simulink library "xpclib"  (Simulink 6.0)
settings: Solver=ode45  SolverMode=SingleTasking  StartTime=0.0  StopTime=10.0  RelTol=1e-3
values from neighbouring files (symbols this model uses):
  base = get_param( gcb, 'base' )    [maddiamondmm.m]    (also in maddiamondmm32frame.m; maddsmm16at.m; mdadsmm16at.m; mdiortddm64x0.m = hex2dec(addr(3:end)))
  block = find_system(bdroot,                          'FollowLinks', 'on',                          'LookUnderMasks', 'all',                          'MaskType', type )    [mdionipci6527.m]
  count = count + 1    (= 5)    [mdecodestate.m]
  port = get_param( gcb, 'port' )    [mdionipci6527.m]    (also in mdiortddm64x0.m = get_param(blocks{i}, 'port'))
undefined symbols (not defined in the file or in its folder): CIO, devid, DIO24, genixlib, get, handlers, irq, mbaseserialmask, mbwaudpmc, mdacbpcidas, mdiamondemeraldmask, mgenix, mmodemcontrol, mquamask, mrs232, msc150checks, mtargetboxleds, mtargetboxwatchdog, mxpccan, PCI, sizeof, vendid
libraries: xpclib x384, simulink x6
(part 1 of 7)
settings Model: RequirementInfo=9  CovMetricSettings=d  Creator=mvetsch  LastModifiedBy=gweast  ProdHWDeviceType=Specified  xpc_rtwmakecfg_data=_xpcaudpmc_
settings Model: ForwardingTableString=|
  | ||__slOldName__||xpclib/A//D/Advantech/PCL-1800 ||__slNewName__||xpcadvantechlib/A//D/PCL-1800 ||__slOldName__||xpclib/A//D/Advantech/PCL-711B||__slNewName__||xpcadvantechlib/A//D/PCL-711B||__slOldName__||xpclib/A//D/Advantech/PCL-812||__slNewName__||xpcadvantechlib/A//D/PCL-812||__slOldName__||xpclib/A//D/Advantech/PCL-812PG||__slNewName__||xpcadvantechlib/A//D/PCL-812PG||__slOldName__||xpclib/A//D/Advantech/PCL-818 ||__slNewName__||xpcadvantechlib/A//D/PCL-818 ||__slOldName__||xpclib/A//D/Advantech/PCL-818H ||__slNewName__||xpcadvantechlib/A//D/PCL-818H ||__slOldName__||xpclib/A//D/Advantech/PCL-818HD ||__slNewName__||xpcadvantechlib/A//D/PCL-818HD ||__slOldName__||xpclib/A//D/Advantech/PCL-818HG ||__slNewName__||xpcadvantechlib/A//D/PCL-818HG ||__slOldName__||xpclib/A//D/Advantech/PCL-818L ||__slNewName__||xpcadvantechlib/A//D/PCL-818L ||__slOldName__||xpclib/A//D/Analogic/AIM12 ||__slNewName__||xpcanalogiclib/A//D/AIM12 ||__slOldName__||xpclib/A//D/Analogic/AIM16 ||__slNewName__||xpcanalogiclib/A//D/AIM16 ||__slOldName__||xpclib/A//D/Burr-Brown/PCI-20019M ||__slNewName__||xpcobsoletelib/Burr-Brown/A//D/PCI-20019M ||__slOldName__||xpclib/A//D/Burr-Brown/PCI-20023M ||__slNewName__||xpcobsoletelib/Burr-Brown/A//D/PCI-20023M ||__slOldName__||xpclib/A//D/Burr-Brown/PCI-20098C ||__slNewName__||xpcobsoletelib/Burr-Brown/A//D/PCI-20098C ||__slOldName__||xpclib/A//D/Computer
  | Boards/CIO-DAS16 JR ||__slNewName__||xpcmeasurementcomputinglib/A//D/CIO-DAS16 JR ||__slOldName__||xpclib/A//D/Computer
  | Boards/CIO-DAS1601 12 ||__slNewName__||xpcmeasurementcomputinglib/A//D/CIO-DAS1601 12 ||__slOldName__||xpclib/A//D/Computer
  | Boards/CIO-DAS1602 12 ||__slNewName__||xpcmeasurementcomputinglib/A//D/CIO-DAS1602 12 ||__slOldName__||xpclib/A//D/Computer
  | Boards/CIO-DAS16 330 ||__slNewName__||xpcmeasurementcomputinglib/A//D/CIO-DAS16 330 ||__slOldName__||xpclib/A//D/Computer
  | Boards/CIO-DAS16JR EXP ||__slNewName__||xpcmeasurementcomputinglib/A//D/CIO-DAS16JR EXP ||__slOldName__||xpclib/A//D/Computer
  | Boards/CIO-DAS16JR 16 ||__slNewName__||xpcmeasurementcomputinglib/A//D/CIO-DAS16JR 16 ||__slOldName__||xpclib/A//D/Computer
  | Boards/CIO-DAS1602 16 ||__slNewName__||xpcmeasurementcomputinglib/A//D/CIO-DAS1602 16 ||__slOldName__||xpclib/A//D/Computer
  | Boards/PC104-DAS16JR 12 ||__slNewName__||xpcmeasurementcomputinglib/A//D/PC104-DAS16JR 12 ||__slOldName__||xpclib/A//D/Computer
  | Boards/PC104-DAS16JR 16 ||__slNewName__||xpcmeasurementcomputinglib/A//D/PC104-DAS16JR 16 ||__slOldName__||xpclib/A//D/Computer
  | Boards/PCI-DAS1200 JR ||__slNewName__||xpcmeasurementcomputinglib/A//D/PCI-DAS1200 JR ||__slOldName__||xpclib/A//D/Computer
  | Boards/PCI-DAS1200 ||__slNewName__||xpcmeasurementcomputinglib/A//D/PCI-DAS1200 ||__slOldName__||xpclib/A//D/Computer
  | Boards/PCI-DAS1602 12 ||__slNewName__||xpcmeasurementcomputinglib/A//D/PCI-DAS1602 12 ||__slOldName__||xpclib/A//D/Computer
  | Boards/PCI-DAS1602 16 ||__slNewName__||xpcmeasurementcomputinglib/A//D/PCI-DAS1602 16 ||__slOldName__||xpclib/A//D/Computer
  | Boards/PCIM-DAS1602 16 ||__slNewName__||xpcmeasurementcomputinglib/A//D/PCIM-DAS1602 16 ||__slOldName__||xpclib/A//D/Contec/AD12-16 ||__slNewName__||xpcconteclib/A//D/AD12-16 ||__slOldName__||xpclib/A//D/Contec/AD12-16E ||__slNewName__||xpcconteclib/A//D/AD12-16E ||__slOldName__||xpclib/A//D/Contec/AD12-16UE ||__slNewName__||xpcconteclib/A//D/AD12-16UE ||__slOldName__||xpclib/A//D/Contec/AD12-64 ||__slNewName__||xpcconteclib/A//D/AD12-64 ||__slOldName__||xpclib/A//D/Contec/AD16-16E ||__slNewName__||xpcconteclib/A//D/AD16-16E ||__slOldName__||xpclib/A//D/Data
  | Translation/DT2821 ||__slNewName__||xpcdatatranslationlib/A//D/DT2821 ||__slOldName__||xpclib/A//D/Data
  | Translation/DT2821-F-16SE ||__slNewName__||xpcdatatranslationlib/A//D/DT2821-F-16SE ||__slOldName__||xpclib/A//D/Data
  | Translation/DT2821-F-8DI ||__slNewName__||xpcdatatranslationlib/A//D/DT2821-F-8DI ||__slOldName__||xpclib/A//D/Data
  | Translation/DT2821-G-16SE ||__slNewName__||xpcdatatranslationlib/A//D/DT2821-G-16SE ||__slOldName__||xpclib/A//D/Data
  | Translation/DT2821-G-8DI ||__slNewName__||xpcdatatranslationlib/A//D/DT2821-G-8DI ||__slOldName__||xpclib/A//D/Data
  | Translation/DT2823 ||__slNewName__||xpcdatatranslationlib/A//D/DT2823 ||__slOldName__||xpclib/A//D/Data
  | Translation/DT2824-PGH ||__slNewName__||xpcdatatranslationlib/A//D/DT2824-PGH ||__slOldName__||xpclib/A//D/Data
  | Translation/DT2824-PGL ||__slNewName__||xpcdatatranslationlib/A//D/DT2824-PGL ||__slOldName__||xpclib/A//D/Data
  | Translation/DT2825 ||__slNewName__||xpcdatatranslationlib/A//D/DT2825 ||__slOldName__||xpclib/A//D/Data
  | Translation/DT2827 ||__slNewName__||xpcdatatranslationlib/A//D/DT2827 ||__slOldName__||xpclib/A//D/Data
  | Translation/DT2828 ||__slNewName__||xpcdatatranslationlib/A//D/DT2828 ||__slOldName__||xpclib/A//D/Diamond/MM ||__slNewName__||xpcdiamondlib/A//D/MM ||__slOldName__||xpclib/A//D/Diamond/MM-16-AT ||__slNewName__||xpcdiamondlib/A//D/MM-16-AT ||__slOldName__||xpclib/A//D/Diamond/MM-32 ||__slNewName__||xpcdiamondlib/A//D/MM-32 ||__slOldName__||xpclib/A//D/Diamond/Prometheus ||__slNewName__||xpcdiamondlib/A//D/Prometheus ||__slOldName__||xpclib/A//D/General
  | Standards/ADADIO ||__slNewName__||xpcgeneralstandardslib/A//D/ADADIO ||__slOldName__||xpclib/A//D/General
  | Standards/ADADIO 1||__slNewName__||xpcgeneralstandardslib/A//D/ADADIO 1||__slOldName__||xpclib/A//D/General
  | Standards/Create Enable Signal||__slNewName__||xpcgeneralstandardslib/A//D/Create Enable Signal||__slOldName__||xpclib/A//D/Gespac/GESADA-1 ||__slNewName__||xpcobsoletelib/Gespac/A//D/GESADA-1 ||__slOldName__||xpclib/A//D/Humusoft/AD 512 ||__slNewName__||xpchumusoftlib/A//D/AD 512 ||__slOldName__||xpclib/A//D/Keithley
  | Metrabyte/KPCI-1801HC ||__slNewName__||xpckeithleylib/A//D/KPCI-1801HC ||__slOldName__||xpclib/A//D/Keithley
  | Metrabyte/KPCI-1802HC ||__slNewName__||xpckeithleylib/A//D/KPCI-1802HC ||__slOldName__||xpclib/A//D/Keithley
  | Metrabyte/DAS-1800HR ||__slNewName__||xpckeithleylib/A//D/DAS-1800HR ||__slOldName__||xpclib/A//D/National
  | Instruments/PCI-6023E ||__slNewName__||xpcnilib/A//D/PCI-6023E ||__slOldName__||xpclib/A//D/National
  | Instruments/PCI-6024E ||__slNewName__||xpcnilib/A//D/PCI-6024E ||__slOldName__||xpclib/A//D/National
  | Instruments/PCI-6025E ||__slNewName__||xpcnilib/A//D/PCI-6025E ||__slOldName__||xpclib/A//D/National
  | Instruments/PCI-6031E ||__slNewName__||xpcnilib/A//D/PCI-6031E ||__slOldName__||xpclib/A//D/National
  | Instruments/PCI-6052E ||__slNewName__||xpcnilib/A//D/PCI-6052E ||__slOldName__||xpclib/A//D/National
  | Instruments/PCI-6071E ||__slNewName__||xpcnilib/A//D/PCI-6071E ||__slOldName__||xpclib/A//D/National
  | Instruments/PCI-MIO-16E-1 ||__slNewName__||xpcnilib/A//D/PCI-6070E ||__slOldName__||xpclib/A//D/National
  | Instruments/PCI-MIO-16E-4 ||__slNewName__||xpcnilib/A//D/PCI-6040E ||__slOldName__||xpclib/A//D/National
  | Instruments/PCI-MIO-16XE-10 ||__slNewName__||xpcnilib/A//D/PCI-6030E ||__slOldName__||xpclib/A//D/National
  | Instruments/PXI-6040E ||__slNewName__||xpcnilib/A//D/PXI-6040E ||__slOldName__||xpclib/A//D/National
  | Instruments/PXI-6070E ||__slNewName__||xpcnilib/A//D/PXI-6070E ||__slOldName__||xpclib/A//D/National
  | Instruments/PXI-6071E ||__slNewName__||xpcnilib/A//D/PXI-6071E ||__slOldName__||xpclib/A//D/Quanser/Q8 ||__slNewName__||xpcquanserlib/A//D/Q8 ||__slOldName__||xpclib/A//D/Real Time
  | Devices/DM6420 ||__slNewName__||xpcrealtimedeviceslib/A//D/DM6420 ||__slOldName__||xpclib/A//D/Real Time
  | Devices/DM6430 ||__slNewName__||xpcrealtimedeviceslib/A//D/DM6430 ||__slOldName__||xpclib/A//D/Real Time
  | Devices/DM7420 ||__slNewName__||xpcrealtimedeviceslib/A//D/DM7420 ||__slOldName__||xpclib/A//D/SBS
  | Technologies/IP-16ADC ||__slNewName__||xpcsbstechnologieslib/A//D/IP-16ADC ||__slOldName__||xpclib/A//D/SBS
  | Technologies/IP-HiADC ||__slNewName__||xpcsbstechnologieslib/A//D/IP-HiADC ||__slOldName__||xpclib/A//D/UEI/PD2-MF 12bit series ||__slNewName__||xpcueilib/A//D/PD2-MF 12bit series ||__slOldName__||xpclib/A//D/UEI/PD2-MF 14bit series ||__slNewName__||xpcueilib/A//D/PD2-MF 14bit series ||__slOldName__||xpclib/A//D/UEI/PD2-MF 16bit series ||__slNewName__||xpcueilib/A//D/PD2-MF 16bit series ||__slOldName__||xpclib/A//D/UEI/PD2-MFS 12bit series ||__slNewName__||xpcueilib/A//D/PD2-MFS 12bit series ||__slOldName__||xpclib/A//D/UEI/PD2-MFS 14bit series ||__slNewName__||xpcueilib/A//D/PD2-MFS 14bit series ||__slOldName__||xpclib/A//D/UEI/PD2-MFS 16bit series ||__slNewName__||xpcueilib/A//D/PD2-MFS 16bit series ||__slOldName__||xpclib/A//D/UEI/PDXI-MF 12bit series ||__slNewName__||xpcueilib/A//D/PDXI-MF 12bit series ||__slOldName__||xpclib/A//D/UEI/PDXI-MF 14bit series ||__slNewName__||xpcueilib/A//D/PDXI-MF 14bit series ||__slOldName__||xpclib/A//D/UEI/PDXI-MF 16bit series ||__slNewName__||xpcueilib/A//D/PDXI-MF 16bit series ||__slOldName__||xpclib/A//D/UEI/PDXI-MFS 12bit series ||__slNewName__||xpcueilib/A//D/PDXI-MFS 12bit series ||__slOldName__||xpclib/A//D/UEI/PDXI-MFS 14bit series ||__slNewName__||xpcueilib/A//D/PDXI-MFS 14bit series ||__slOldName__||xpclib/A//D/UEI/PDXI-MFS 16bit series ||__slNewName__||xpcueilib/A//D/PDXI-MFS 16bit series ||__slOldName__||xpclib/A//D/Versalogic/VSBC-6 ||__slNewName__||xpcversalogiclib/A//D/VSBC-6 ||__slOldName__||xpclib/A//D
  | Frame/Diamond/MM-32 Frame ||__slNewName__||xpcdiamondlib/A//D
  | Frame/MM-32 Frame ||__slOldName__||xpclib/A//D
  | Frame/UEI/PD2-MF Frame 12bit series ||__slNewName__||xpcueilib/A//D
  | Frame/PD2-MF Frame 12bit series ||__slOldName__||xpclib/A//D
  | Frame/UEI/PD2-MF Frame 14bit series ||__slNewName__||xpcueilib/A//D
  | Frame/PD2-MF Frame 14bit series ||__slOldName__||xpclib/A//D
  | Frame/UEI/PD2-MF Frame 16bit series ||__slNewName__||xpcueilib/A//D
  | Frame/PD2-MF Frame 16bit series ||__slOldName__||xpclib/A//D
  | Frame/UEI/PD2-MFS Frame 12bit series ||__slNewName__||xpcueilib/A//D
  | Frame/PD2-MFS Frame 12bit series ||__slOldName__||xpclib/A//D
  | Frame/UEI/PD2-MFS Frame 14bit series ||__slNewName__||xpcueilib/A//D
  | Frame/PD2-MFS Frame 14bit series ||__slOldName__||xpclib/A//D
  | Frame/UEI/PD2-MFS Frame 16bit series ||__slNewName__||xpcueilib/A//D
  | Frame/PD2-MFS Frame 16bit series ||__slOldName__||xpclib/A//D
  | Frame/UEI/PDXI-MF Frame 12bit series ||__slNewName__||xpcueilib/A//D
  | Frame/PDXI-MF Frame 12bit series ||__slOldName__||xpclib/A//D
  | Frame/UEI/PDXI-MF Frame 14bit series ||__slNewName__||xpcueilib/A//D
  | Frame/PDXI-MF Frame 14bit series ||__slOldName__||xpclib/A//D
  | Frame/UEI/PDXI-MF Frame 16bit series ||__slNewName__||xpcueilib/A//D
  | Frame/PDXI-MF Frame 16bit series ||__slOldName__||xpclib/A//D
  | Frame/UEI/PDXI-MFS Frame 12bit series ||__slNewName__||xpcueilib/A//D
  | Frame/PDXI-MFS Frame 12bit series ||__slOldName__||xpclib/A//D
  | Frame/UEI/PDXI-MFS Frame 14bit series ||__slNewName__||xpcueilib/A//D
  | Frame/PDXI-MFS Frame 14bit series ||__slOldName__||xpclib/A//D
  | Frame/UEI/PDXI-MFS Frame 16bit series ||__slNewName__||xpcueilib/A//D
  | Frame/PDXI-MFS Frame 16bit series ||__slOldName__||xpclib/D//A/Advantech/PCL-711B||__slNewName__||xpcadvantechlib/D//A/PCL-711B ||__slOldName__||xpclib/D//A/Advantech/PCL-812||__slNewName__||xpcadvantechlib/D//A/PCL-812 ||__slOldName__||xpclib/D//A/Advantech/PCL-812PG||__slNewName__||xpcadvantechlib/D//A/PCL-812PG ||__slOldName__||xpclib/D//A/Advantech/PCL-818 ||__slNewName__||xpcadvantechlib/D//A/PCL-818 ||__slOldName__||xpclib/D//A/Advantech/PCL-818L ||__slNewName__||xpcadvantechlib/D//A/PCL-818L ||__slOldName__||xpclib/D//A/Advantech/PCL-818HG ||__slNewName__||xpcadvantechlib/D//A/PCL-818HG ||__slOldName__||xpclib/D//A/Advantech/PCL-818H ||__slNewName__||xpcadvantechlib/D//A/PCL-818H ||__slOldName__||xpclib/D//A/Advantech/PCL-818HD ||__slNewName__||xpcadvantechlib/D//A/PCL-818HD ||__slOldName__||xpclib/D//A/Advantech/PCL-1800 ||__slNewName__||xpcadvantechlib/D//A/PCL-1800 ||__slOldName__||xpclib/D//A/Advantech/PCL-726 ||__slNewName__||xpcadvantechlib/D//A/PCL-726 ||__slOldName__||xpclib/D//A/Advantech/PCL-727 ||__slNewName__||xpcadvantechlib/D//A/PCL-727 ||__slOldName__||xpclib/D//A/Advantech/PCL-728 ||__slNewName__||xpcadvantechlib/D//A/PCL-728 ||__slOldName__||xpclib/D//A/Burr-Brown/PCI-20003M ||__slNewName__||xpcobsoletelib/Burr-Brown/D//A/PCI-20003M ||__slOldName__||xpclib/D//A/Computer
  | Boards/CIO-DAS1601 12 ||__slNewName__||xpcmeasurementcomputinglib/D//A/CIO-DAS1601 12 ||__slOldName__||xpclib/D//A/Computer
  | Boards/CIO-DAS1602 12 ||__slNewName__||xpcmeasurementcomputinglib/D//A/CIO-DAS1602 12 ||__slOldName__||xpclib/D//A/Computer
  | Boards/CIO-DAS1602 16 ||__slNewName__||xpcmeasurementcomputinglib/D//A/CIO-DAS1602 16 ||__slOldName__||xpclib/D//A/Computer
  | Boards/CIO-DDA06 ||__slNewName__||xpcmeasurementcomputinglib/D//A/CIO-DDA06 ||__slOldName__||xpclib/D//A/Computer
  | Boards/CIO-DAC08 ||__slNewName__||xpcmeasurementcomputinglib/D//A/CIO-DAC08 ||__slOldName__||xpclib/D//A/Computer
  | Boards/CIO-DAC16 ||__slNewName__||xpcmeasurementcomputinglib/D//A/CIO-DAC16 ||__slOldName__||xpclib/D//A/Computer
  | Boards/PC104-DAC06 ||__slNewName__||xpcmeasurementcomputinglib/D//A/PC104-DAC06 ||__slOldName__||xpclib/D//A/Computer
  | Boards/CIO-DDA06 16 ||__slNewName__||xpcmeasurementcomputinglib/D//A/CIO-DDA06 16 ||__slOldName__||xpclib/D//A/Computer
  | Boards/CIO-DAC08 16 ||__slNewName__||xpcmeasurementcomputinglib/D//A/CIO-DAC08 16 ||__slOldName__||xpclib/D//A/Computer
  | Boards/CIO-DAC16 16 ||__slNewName__||xpcmeasurementcomputinglib/D//A/CIO-DAC16 16 ||__slOldName__||xpclib/D//A/Computer
  | Boards/PCI-DAS1200 ||__slNewName__||xpcmeasurementcomputinglib/D//A/PCI-DAS1200 ||__slOldName__||xpclib/D//A/Computer
  | Boards/PCI-DAS1602 12 ||__slNewName__||xpcmeasurementcomputinglib/D//A/PCI-DAS1602 12 ||__slOldName__||xpclib/D//A/Computer
  | Boards/PCI-DAS1602 16 ||__slNewName__||xpcmeasurementcomputinglib/D//A/PCI-DAS1602 16 ||__slOldName__||xpclib/D//A/Computer
  | Boards/PCIM-DAS1602 16 ||__slNewName__||xpcmeasurementcomputinglib/D//A/PCIM-DAS1602 16 ||__slOldName__||xpclib/D//A/Computer
  | Boards/PCI-DDA02 12 ||__slNewName__||xpcmeasurementcomputinglib/D//A/PCI-DDA02 12 ||__slOldName__||xpclib/D//A/Computer
  | Boards/PCI-DDA04 12 ||__slNewName__||xpcmeasurementcomputinglib/D//A/PCI-DDA04 12 ||__slOldName__||xpclib/D//A/Computer
  | Boards/PCI-DDA08 12 ||__slNewName__||xpcmeasurementcomputinglib/D//A/PCI-DDA08 12 ||__slOldName__||xpclib/D//A/Computer
  | Boards/PCI-DDA02 16 ||__slNewName__||xpcmeasurementcomputinglib/D//A/PCI-DDA02 16 ||__slOldName__||xpclib/D//A/Computer
  | Boards/PCI-DDA04 16 ||__slNewName__||xpcmeasurementcomputinglib/D//A/PCI-DDA04 16 ||__slOldName__||xpclib/D//A/Computer
  | Boards/PCI-DDA08 16 ||__slNewName__||xpcmeasurementcomputinglib/D//A/PCI-DDA08 16 ||__slOldName__||xpclib/D//A/Computer
  | Boards/PCIM-DDA06 16 ||__slNewName__||xpcmeasurementcomputinglib/D//A/PCIM-DDA06 16 ||__slOldName__||xpclib/D//A/Contec/DA12-4 ||__slNewName__||xpcconteclib/D//A/DA12-4 ||__slOldName__||xpclib/D//A/Contec/DA12-16 ||__slNewName__||xpcconteclib/D//A/DA12-16 ||__slOldName__||xpclib/D//A/Contec/AD12-16E ||__slNewName__||xpcconteclib/D//A/AD12-16E ||__slOldName__||xpclib/D//A/Contec/AD12-16UE  ||__slNewName__||xpcconteclib/D//A/AD12-16UE ||__slOldName__||xpclib/D//A/Contec/AD16-16E  ||__slNewName__||xpcconteclib/D//A/AD16-16E ||__slOldName__||xpclib/D//A/Data
  | Translation/DT2821 ||__slNewName__||xpcdatatranslationlib/D//A/DT2821 ||__slOldName__||xpclib/D//A/Data
  | Translation/DT2821-F-16SE ||__slNewName__||xpcdatatranslationlib/D//A/DT2821-F-16SE ||__slOldName__||xpclib/D//A/Data
  | Translation/DT2821-F-8DI ||__slNewName__||xpcdatatranslationlib/D//A/DT2821-F-8DI ||__slOldName__||xpclib/D//A/Data
  | Translation/DT2821-G-16SE ||__slNewName__||xpcdatatranslationlib/D//A/DT2821-G-16SE ||__slOldName__||xpclib/D//A/Data
  | Translation/DT2821-G-8DI ||__slNewName__||xpcdatatranslationlib/D//A/DT2821-G-8DI ||__slOldName__||xpclib/D//A/Data
  | Translation/DT2823 ||__slNewName__||xpcdatatranslationlib/D//A/DT2823 ||__slOldName__||xpclib/D//A/Data
  | Translation/DT2825 ||__slNewName__||xpcdatatranslationlib/D//A/DT2825 ||__slOldName__||xpclib/D//A/Data
  | Translation/DT2827 ||__slNewName__||xpcdatatranslationlib/D//A/DT2827 ||__slOldName__||xpclib/D//A/Data
  | Translation/DT2828 ||__slNewName__||xpcdatatranslationlib/D//A/DT2828 ||__slOldName__||xpclib/D//A/Diamond/Ruby-MM ||__slNewName__||xpcdiamondlib/D//A/Ruby-MM ||__slOldName__||xpclib/D//A/Diamond/Ruby-MM-416 ||__slNewName__||xpcdiamondlib/D//A/Ruby-MM-416 ||__slOldName__||xpclib/D//A/Diamond/Ruby-MM-1612 ||__slNewName__||xpcdiamondlib/D//A/Ruby-MM-1612 ||__slOldName__||xpclib/D//A/Diamond/MM ||__slNewName__||xpcdiamondlib/D//A/MM ||__slOldName__||xpclib/D//A/Diamond/MM-32 ||__slNewName__||xpcdiamondlib/D//A/MM-32 ||__slOldName__||xpclib/D//A/Diamond/Prometheus ||__slNewName__||xpcdiamondlib/D//A/Prometheus ||__slOldName__||xpclib/D//A/Diamond/MM-16-AT ||__slNewName__||xpcdiamondlib/D//A/MM-16-AT ||__slOldName__||xpclib/D//A/General
  | Standards/ADADIO ||__slNewName__||xpcgeneralstandardslib/D//A/ADADIO ||__slOldName__||xpclib/D//A/General
  | Standards/Create Enable Signal||__slNewName__||xpcgeneralstandardslib/D//A/Create Enable Signal||__slOldName__||xpclib/D//A/General
  | Standards/ADADIO 1||__slNewName__||xpcgeneralstandardslib/D//A/ADADIO 1||__slOldName__||xpclib/D//A/General
  | Standards/PMC-16AO-12 ||__slNewName__||xpcgeneralstandardslib/D//A/PMC-16AO-12 ||__slOldName__||xpclib/D//A/Gespac/GESADA-1 ||__slNewName__||xpcobsoletelib/Gespac/D//A/GESADA-1 ||__slOldName__||xpclib/D//A/Humusoft/AD 512 ||__slNewName__||xpchumusoftlib/D//A/AD 512 ||__slOldName__||xpclib/D//A/Keithley
  | Metrabyte/KPCI-1801HC ||__slNewName__||xpckeithleylib/D//A/KPCI-1801HC ||__slOldName__||xpclib/D//A/Keithley
  | Metrabyte/KPCI-1802HC ||__slNewName__||xpckeithleylib/D//A/KPCI-1802HC ||__slOldName__||xpclib/D//A/National
  | Instruments/AT-AO-6 ||__slNewName__||xpcnilib/D//A/AT-AO-6 ||__slOldName__||xpclib/D//A/National
  | Instruments/AT-AO-10 ||__slNewName__||xpcnilib/D//A/AT-AO-10 ||__slOldName__||xpclib/D//A/National
  | Instruments/PCI-6703 ||__slNewName__||xpcnilib/D//A/PCI-6703 ||__slOldName__||xpclib/D//A/National
  | Instruments/PXI-6071E ||__slNewName__||xpcnilib/D//A/PXI-6071E ||__slOldName__||xpclib/D//A/National
  | Instruments/PCI-6024E ||__slNewName__||xpcnilib/D//A/PCI-6024E ||__slOldName__||xpclib/D//A/National
  | Instruments/PCI-6025E ||__slNewName__||xpcnilib/D//A/PCI-6025E ||__slOldName__||xpclib/D//A/National
  | Instruments/PCI-6704 ||__slNewName__||xpcnilib/D//A/PCI-6704 ||__slOldName__||xpclib/D//A/National
  | Instruments/PXI-6704 ||__slNewName__||xpcnilib/D//A/PXI-6704 ||__slOldName__||xpclib/D//A/National
  | Instruments/PCI-MIO-16E-1 ||__slNewName__||xpcnilib/D//A/PCI-6070E ||__slOldName__||xpclib/D//A/National
  | Instruments/PCI-MIO-16E-4 ||__slNewName__||xpcnilib/D//A/PCI-6040E ||__slOldName__||xpclib/D//A/National
  | Instruments/PXI-6070E ||__slNewName__||xpcnilib/D//A/PXI-6070E ||__slOldName__||xpclib/D//A/National
  | Instruments/PXI-6040E ||__slNewName__||xpcnilib/D//A/PXI-6040E ||__slOldName__||xpclib/D//A/National
  | Instruments/PCI-6071E ||__slNewName__||xpcnilib/D//A/PCI-6071E ||__slOldName__||xpclib/D//A/National
  | Instruments/PCI-6052E ||__slNewName__||xpcnilib/D//A/PCI-6052E ||__slOldName__||xpclib/D//A/National
  | Instruments/PCI-MIO-16XE-10 ||__slNewName__||xpcnilib/D//A/PCI-6030E ||__slOldName__||xpclib/D//A/National
  | Instruments/PCI-6031E ||__slNewName__||xpcnilib/D//A/PCI-6031E ||__slOldName__||xpclib/D//A/National
  | Instruments/PCI-6713 ||__slNewName__||xpcnilib/D//A/PCI-6713 ||__slOldName__||xpclib/D//A/National
  | Instruments/PXI-6713 ||__slNewName__||xpcnilib/D//A/PXI-6713 ||__slOldName__||xpclib/D//A/National
  | Instruments/PCI-6713 1||__slNewName__||xpcnilib/D//A/PCI-6713 1 ||__slOldName__||xpclib/D//A/Real Time
  | Devices/DM6420 ||__slNewName__||xpcrealtimedeviceslib/D//A/DM6420 ||__slOldName__||xpclib/D//A/Real Time
  | Devices/DM6430 ||__slNewName__||xpcrealtimedeviceslib/D//A/DM6430 ||__slOldName__||xpclib/D//A/Real Time
  | Devices/DM6604 ||__slNewName__||xpcrealtimedeviceslib/D//A/DM6604 ||__slOldName__||xpclib/D//A/SBS
  | Technologies/IP-DAC ||__slNewName__||xpcsbstechnologieslib/D//A/IP-DAC ||__slOldName__||xpclib/D//A/SBS
  | Technologies/IP-16DAC ||__slNewName__||xpcsbstechnologieslib/D//A/IP-16DAC ||__slOldName__||xpclib/D//A/UEI/PD2-MF 12bit series ||__slNewName__||xpcueilib/D//A/PD2-MF 12bit series||__slOldName__||xpclib/D//A/UEI/PD2-MFS 12bit series ||__slNewName__||xpcueilib/D//A/PD2-MFS 12bit series||__slOldName__||xpclib/D//A/UEI/PDXI-MF 12bit series ||__slNewName__||xpcueilib/D//A/PDXI-MF 12bit series||__slOldName__||xpclib/D//A/UEI/PDXI-MFS 12bit series ||__slNewName__||xpcueilib/D//A/PDXI-MFS 12bit series||__slOldName__||xpclib/D//A/UEI/PD2-MF 14bit series ||__slNewName__||xpcueilib/D//A/PD2-MF 14bit series||__slOldName__||xpclib/D//A/UEI/PD2-MFS 14bit series ||__slNewName__||xpcueilib/D//A/PD2-MFS 14bit series||__slOldName__||xpclib/D//A/UEI/PDXI-MF 14bit series ||__slNewName__||xpcueilib/D//A/PDXI-MF 14bit series||__slOldName__||xpclib/D//A/UEI/PDXI-MFS 14bit series ||__slNewName__||xpcueilib/D//A/PDXI-MFS 14bit series||__slOldName__||xpclib/D//A/UEI/PD2-MF 16bit series ||__slNewName__||xpcueilib/D//A/PD2-MF 16bit series||__slOldName__||xpclib/D//A/UEI/PD2-MFS 16bit series ||__slNewName__||xpcueilib/D//A/PD2-MFS 16bit series||__slOldName__||xpclib/D//A/UEI/PDXI-MF 16bit series ||__slNewName__||xpcueilib/D//A/PDXI-MF 16bit series||__slOldName__||xpclib/D//A/UEI/PDXI-MFS 16bit series ||__slNewName__||xpcueilib/D//A/PDXI-MFS 16bit series||__slOldName__||xpclib/D//A/UEI/PD2-AO series ||__slNewName__||xpcueilib/D//A/PD2-AO series||__slOldName__||xpclib/D//A/UEI/PDXI-AO series ||__slNewName__||xpcueilib/D//A/PDXI-AO series||__slOldName__||xpclib/Digital
  | Input/Advantech/PCL-711B||__slNewName__||xpcadvantechlib/Digital
  | Input/PCL-711B ||__slOldName__||xpclib/Digital
  | Input/Advantech/PCL-812||__slNewName__||xpcadvantechlib/Digital
  | Input/PCL-812 ||__slOldName__||xpclib/Digital
  | Input/Advantech/PCL-812PG||__slNewName__||xpcadvantechlib/Digital
  | Input/PCL-812PG ||__slOldName__||xpclib/Digital
  | Input/Advantech/PCL-818 ||__slNewName__||xpcadvantechlib/Digital
  | Input/PCL-818 ||__slOldName__||xpclib/Digital
  | Input/Advantech/PCL-818L ||__slNewName__||xpcadvantechlib/Digital
  | Input/PCL-818L ||__slOldName__||xpclib/Digital
  | Input/Advantech/PCL-818HG ||__slNewName__||xpcadvantechlib/Digital
  | Input/PCL-818HG ||__slOldName__||xpclib/Digital
  | Input/Advantech/PCL-818H ||__slNewName__||xpcadvantechlib/Digital
  | Input/PCL-818H ||__slOldName__||xpclib/Digital
  | Input/Advantech/PCL-818HD ||__slNewName__||xpcadvantechlib/Digital
  | Input/PCL-818HD ||__slOldName__||xpclib/Digital
  | Input/Advantech/PCL-1800 ||__slNewName__||xpcadvantechlib/Digital
  | Input/PCL-1800 ||__slOldName__||xpclib/Digital
  | Input/Advantech/PCL-726 ||__slNewName__||xpcadvantechlib/Digital
  | Input/PCL-726 ||__slOldName__||xpclib/Digital
  | Input/Advantech/PCL-727 ||__slNewName__||xpcadvantechlib/Digital
  | Input/PCL-727 ||__slOldName__||xpclib/Digital
  | Input/Analogic/AIM12 ||__slNewName__||xpcanalogiclib/Digital
  | Input/AIM12 ||__slOldName__||xpclib/Digital
  | Input/Analogic/AIM16 ||__slNewName__||xpcanalogiclib/Digital
  | Input/AIM16 ||__slOldName__||xpclib/Digital
  | Input/Burr-Brown/PCI-20041C ||__slNewName__||xpcobsoletelib/Burr-Brown/Digital
  | Input/PCI-20041C ||__slOldName__||xpclib/Digital
  | Input/Burr-Brown/PCI-20098C ||__slNewName__||xpcobsoletelib/Burr-Brown/Digital
  | Input/PCI-20098C ||__slOldName__||xpclib/Digital
  | Input/BVM/PMCDIO64 ||__slNewName__||xpcobsoletelib/BVM/Digital
  | Input/PMCDIO64 ||__slOldName__||xpclib/Digital
  | Input/Computer
  | Boards/CIO-DDA06 ||__slNewName__||xpcmeasurementcomputinglib/Digital
  | Input/CIO-DDA06 ||__slOldName__||xpclib/Digital
  | Input/Computer
  | Boards/CIO-DDA06//16 ||__slNewName__||xpcmeasurementcomputinglib/Digital
  | Input/CIO-DDA06//16 ||__slOldName__||xpclib/Digital
  | Input/Computer
  | Boards/CIO-DAS1601 12 ||__slNewName__||xpcmeasurementcomputinglib/Digital
  | Input/CIO-DAS1601 12 ||__slOldName__||xpclib/Digital
  | Input/Computer
  | Boards/CIO-DAS1602 12 ||__slNewName__||xpcmeasurementcomputinglib/Digital
  | Input/CIO-DAS1602 12 ||__slOldName__||xpclib/Digital
  | Input/Computer
  | Boards/CIO-DAS1602 16 ||__slNewName__||xpcmeasurementcomputinglib/Digital
  | Input/CIO-DAS1602 16 ||__slOldName__||xpclib/Digital
  | Input/Computer
  | Boards/CIO-DIO24 ||__slNewName__||xpcmeasurementcomputinglib/Digital
  | Input/CIO-DIO24 ||__slOldName__||xpclib/Digital
  | Input/Computer
  | Boards/CIO-DIO48 ||__slNewName__||xpcmeasurementcomputinglib/Digital
  | Input/CIO-DIO48 ||__slOldName__||xpclib/Digital
  | Input/Computer
  | Boards/CIO-DIO96 ||__slNewName__||xpcmeasurementcomputinglib/Digital
  | Input/CIO-DIO96 ||__slOldName__||xpclib/Digital
  | Input/Computer
  | Boards/CIO-DIO192 ||__slNewName__||xpcmeasurementcomputinglib/Digital
  | Input/CIO-DIO192 ||__slOldName__||xpclib/Digital
  | Input/Computer
  | Boards/CIO-DIO24H ||__slNewName__||xpcmeasurementcomputinglib/Digital
  | Input/CIO-DIO24H ||__slOldName__||xpclib/Digital
  | Input/Computer
  | Boards/CIO-DIO48H ||__slNewName__||xpcmeasurementcomputinglib/Digital
  | Input/CIO-DIO48H ||__slOldName__||xpclib/Digital
  | Input/Computer
  | Boards/CIO-PDISO16 ||__slNewName__||xpcmeasurementcomputinglib/Digital
  | Input/CIO-PDISO16 ||__slOldName__||xpclib/Digital
  | Input/Computer
  | Boards/PC104-DAS16JR 12 ||__slNewName__||xpcmeasurementcomputinglib/Digital
  | Input/PC104-DAS16JR 12 ||__slOldName__||xpclib/Digital
  | Input/Computer
  | Boards/PC104-DAS16JR 16 ||__slNewName__||xpcmeasurementcomputinglib/Digital
  | Input/PC104-DAS16JR 16 ||__slOldName__||xpclib/Digital
  | Input/Computer
  | Boards/PC104-DIO48 ||__slNewName__||xpcmeasurementcomputinglib/Digital
  | Input/PC104-DIO48 ||__slOldName__||xpclib/Digital
  | Input/Computer
  | Boards/PCI-DAS1200 ||__slNewName__||xpcmeasurementcomputinglib/Digital
  | Input/PCI-DAS1200 ||__slOldName__||xpclib/Digital
  | Input/Computer
  | Boards/PCI-DAS1200 JR ||__slNewName__||xpcmeasurementcomputinglib/Digital
  | Input/PCI-DAS1200 JR ||__slOldName__||xpclib/Digital
  | Input/Computer
  | Boards/PCI-DAS1602 12 ||__slNewName__||xpcmeasurementcomputinglib/Digital
  | Input/PCI-DAS1602 12 ||__slOldName__||xpclib/Digital
  | Input/Computer
  | Boards/PCI-DAS1602 16 ||__slNewName__||xpcmeasurementcomputinglib/Digital
  | Input/PCI-DAS1602 16 ||__slOldName__||xpclib/Digital
  | Input/Computer
  | Boards/PCIM-DAS1602 16 ||__slNewName__||xpcmeasurementcomputinglib/Digital
  | Input/PCIM-DAS1602 16 ||__slOldName__||xpclib/Digital
  | Input/Computer
  | Boards/PCI-DIO24 ||__slNewName__||xpcmeasurementcomputinglib/Digital
  | Input/PCI-DIO24 ||__slOldName__||xpclib/Digital
  | Input/Computer
  | Boards/PCI-DIO24H ||__slNewName__||xpcmeasurementcomputinglib/Digital
  | Input/PCI-DIO24H ||__slOldName__||xpclib/Digital
  | Input/Computer
  | Boards/PCI-DIO48H ||__slNewName__||xpcmeasurementcomputinglib/Digital
  | Input/PCI-DIO48H ||__slOldName__||xpclib/Digital
  | Input/Computer
  | Boards/PCI-DIO96 ||__slNewName__||xpcmeasurementcomputinglib/Digital
  | Input/PCI-DIO96 ||__slOldName__||xpclib/Digital
  | Input/Computer
  | Boards/PCI-DIO96H ||__slNewName__||xpcmeasurementcomputinglib/Digital
  | Input/PCI-DIO96H ||__slOldName__||xpclib/Digital
  | Input/Computer
  | Boards/PCI-DDA02 12 ||__slNewName__||xpcmeasurementcomputinglib/Digital
  | Input/PCI-DDA02 12 ||__slOldName__||xpclib/Digital
  | Input/Computer
  | Boards/PCI-DDA04 12 ||__slNewName__||xpcmeasurementcomputinglib/Digital
  | Input/PCI-DDA04 12 ||__slOldName__||xpclib/Digital
  | Input/Computer
  | Boards/PCI-DDA08 12 ||__slNewName__||xpcmeasurementcomputinglib/Digital
  | Input/PCI-DDA08 12 ||__slOldName__||xpclib/Digital
  | Input/Computer
  | Boards/PCI-PDISO8 ||__slNewName__||xpcmeasurementcomputinglib/Digital
  | Input/PCI-PDISO8 ||__slOldName__||xpclib/Digital
  | Input/Computer
  | Boards/PCI-PDISO16 ||__slNewName__||xpcmeasurementcomputinglib/Digital
  | Input/PCI-PDISO16 ||__slOldName__||xpclib/Digital
  | Input/Computer
  | Boards/PCI-DDA02 16 ||__slNewName__||xpcmeasurementcomputinglib/Digital
  | Input/PCI-DDA02 16 ||__slOldName__||xpclib/Digital
  | Input/Computer
  | Boards/PCI-DDA04 16 ||__slNewName__||xpcmeasurementcomputinglib/Digital
  | Input/PCI-DDA04 16 ||__slOldName__||xpclib/Digital
  | Input/Computer
  | Boards/PCI-DDA08 16 ||__slNewName__||xpcmeasurementcomputinglib/Digital
  | Input/PCI-DDA08 16 ||__slOldName__||xpclib/Digital
  | Input/Computer
  | Boards/PCIM-DDA06 16 ||__slNewName__||xpcmeasurementcomputinglib/Digital
  | Input/PCIM-DDA06 16 ||__slOldName__||xpclib/Digital
  | Input/Computer
  | Boards/PCI-DUAL-AC5 ||__slNewName__||xpcmeasurementcomputinglib/Digital
  | Input/PCI-DUAL-AC5 ||__slOldName__||xpclib/Digital
  | Input/Contec/PIO-3232T ||__slNewName__||xpcconteclib/Digital
  | Input/PIO-3232T ||__slOldName__||xpclib/Digital
  | Input/Contec/AD12-16  ||__slNewName__||xpcconteclib/Digital
  | Input/AD12-16 ||__slOldName__||xpclib/Digital
  | Input/Contec/AD12-64 ||__slNewName__||xpcconteclib/Digital
  | Input/AD12-64 ||__slOldName__||xpclib/Digital
  | Input/Data
  | Translation/DT2821 ||__slNewName__||xpcdatatranslationlib/Digital
  | Input/DT2821 ||__slOldName__||xpclib/Digital
  | Input/Data
  | Translation/DT2821-F-16SE ||__slNewName__||xpcdatatranslationlib/Digital
  | Input/DT2821-F-16SE ||__slOldName__||xpclib/Digital
  | Input/Data
  | Translation/DT2821-F-8DI ||__slNewName__||xpcdatatranslationlib/Digital
  | Input/DT2821-F-8DI ||__slOldName__||xpclib/Digital
  | Input/Data
  | Translation/DT2821-G-16SE ||__slNewName__||xpcdatatranslationlib/Digital
  | Input/DT2821-G-16SE ||__slOldName__||xpclib/Digital
  | Input/Data
  | Translation/DT2821-G-8DI ||__slNewName__||xpcdatatranslationlib/Digital
  | Input/DT2821-G-8DI ||__slOldName__||xpclib/Digital
  | Input/Data
  | Translation/DT2823 ||__slNewName__||xpcdatatranslationlib/Digital
  | Input/DT2823 ||__slOldName__||xpclib/Digital
  | Input/Data
  | Translation/DT2824-PGH ||__slNewName__||xpcdatatranslationlib/Digital
  | Input/DT2824-PGH ||__slOldName__||xpclib/Digital
  | Input/Data
  | Translation/DT2824-PGL ||__slNewName__||xpcdatatranslationlib/Digital
  | Input/DT2824-PGL ||__slOldName__||xpclib/Digital
  | Input/Data
  | Translation/DT2825 ||__slNewName__||xpcdatatranslationlib/Digital
  | Input/DT2825 ||__slOldName__||xpclib/Digital
  | Input/Data
  | Translation/DT2827 ||__slNewName__||xpcdatatranslationlib/Digital
  | Input/DT2827 ||__slOldName__||xpclib/Digital
  | Input/Data
  | Translation/DT2828 ||__slNewName__||xpcdatatranslationlib/Digital
  | Input/DT2828 ||__slOldName__||xpclib/Digital
  | Input/Diamond/Ruby-MM ||__slNewName__||xpcdiamondlib/Digital
  | Input/Ruby-MM ||__slOldName__||xpclib/Digital
  | Input/Diamond/Ruby-MM-416 ||__slNewName__||xpcdiamondlib/Digital
  | Input/Ruby-MM-416 ||__slOldName__||xpclib/Digital
  | Input/Diamond/Ruby-MM-1612 ||__slNewName__||xpcdiamondlib/Digital
  | Input/Ruby-MM-1612 ||__slOldName__||xpclib/Digital
  | Input/Diamond/QUARTZ-MM-5 ||__slNewName__||xpcdiamondlib/Digital
  | Input/QUARTZ-MM-5 ||__slOldName__||xpclib/Digital
  | Input/Diamond/QUARTZ-MM-10 ||__slNewName__||xpcdiamondlib/Digital
  | Input/QUARTZ-MM-10 ||__slOldName__||xpclib/Digital
  | Input/Diamond/Prometheus ||__slNewName__||xpcdiamondlib/Digital
  | Input/Prometheus||__slOldName__||xpclib/Digital
  | Input/Diamond/MM ||__slNewName__||xpcdiamondlib/Digital
  | Input/MM ||__slOldName__||xpclib/Digital
  | Input/Diamond/MM-32 ||__slNewName__||xpcdiamondlib/Digital
  | Input/MM-32 ||__slOldName__||xpclib/Digital
  | Input/Diamond/MM-16-AT ||__slNewName__||xpcdiamondlib/Digital
  | Input/MM-16-AT ||__slOldName__||xpclib/Digital
  | Input/Diamond/Onyx-MM ||__slNewName__||xpcdiamondlib/Digital
  | Input/Onyx-MM ||__slOldName__||xpclib/Digital
  | Input/Diamond/Onyx-MM-DIO ||__slNewName__||xpcdiamondlib/Digital
  | Input/Onyx-MM-DIO ||__slOldName__||xpclib/Digital
  | Input/Diamond/Garnet-MM ||__slNewName__||xpcdiamondlib/Digital
  | Input/Garnet-MM ||__slOldName__||xpclib/Digital
  | Input/General
  | Standards/ADADIO ||__slNewName__||xpcgeneralstandardslib/Digital
  | Input/ADADIO ||__slOldName__||xpclib/Digital
  | Input/Gespac/GESPIA-2A ||__slNewName__||xpcobsoletelib/Gespac/Digital
  | Input/GESPIA-2A ||__slOldName__||xpclib/Digital
  | Input/Humusoft/AD 512 ||__slNewName__||xpchumusoftlib/Digital
  | Input/AD 512 ||__slOldName__||xpclib/Digital
  | Input/Keithley
  | Metrabyte/KPCI-1801HC ||__slNewName__||xpckeithleylib/Digital
  | Input/KPCI-1801HC ||__slOldName__||xpclib/Digital
  | Input/Keithley
  | Metrabyte/KPCI-1802HC ||__slNewName__||xpckeithleylib/Digital
  | Input/KPCI-1802HC ||__slOldName__||xpclib/Digital
  | Input/Keithley
  | Metrabyte/DAS-1800HR ||__slNewName__||xpckeithleylib/Digital
  | Input/DAS-1800HR ||__slOldName__||xpclib/Digital
  | Input/National
  | Instruments/PC-DIO-24 ||__slNewName__||xpcnilib/Digital
  | Input/PC-DIO-24 ||__slOldName__||xpclib/Digital
  | Input/National
  | Instruments/PC-TIO-10 ||__slNewName__||xpcnilib/Digital
  | Input/PC-TIO-10 ||__slOldName__||xpclib/Digital
  | Input/National
  | Instruments/PCI-6503 ||__slNewName__||xpcnilib/Digital
  | Input/PCI-6503 ||__slOldName__||xpclib/Digital
  | Input/National
  | Instruments/PCI-DIO-96 ||__slNewName__||xpcnilib/Digital
  | Input/PCI-DIO-96 ||__slOldName__||xpclib/Digital
  | Input/National
  | Instruments/PCI-6023E ||__slNewName__||xpcnilib/Digital
  | Input/PCI-6023E ||__slOldName__||xpclib/Digital
  | Input/National
  | Instruments/PCI-6024E ||__slNewName__||xpcnilib/Digital
  | Input/PCI-6024E ||__slOldName__||xpclib/Digital
  | Input/National
  | Instruments/PCI-6025E ||__slNewName__||xpcnilib/Digital
  | Input/PCI-6025E ||__slOldName__||xpclib/Digital
  | Input/National
  | Instruments/PCI-6025E 8255 ||__slNewName__||xpcnilib/Digital
  | Input/PCI-6025E 8255 ||__slOldName__||xpclib/Digital
  | Input/National
  | Instruments/PCI-MIO-16E-1 ||__slNewName__||xpcnilib/Digital
  | Input/PCI-6070E ||__slOldName__||xpclib/Digital
  | Input/National
  | Instruments/PCI-MIO-16E-4 ||__slNewName__||xpcnilib/Digital
  | Input/PCI-6040E ||__slOldName__||xpclib/Digital
  | Input/National
  | Instruments/PCI-6071E ||__slNewName__||xpcnilib/Digital
  | Input/PCI-6071E ||__slOldName__||xpclib/Digital
  | Input/National
  | Instruments/PCI-6527 ||__slNewName__||xpcnilib/Digital
  | Input/PCI-6527 ||__slOldName__||xpclib/Digital
  | Input/National
  | Instruments/PCI-6052E ||__slNewName__||xpcnilib/Digital
  | Input/PCI-6052E ||__slOldName__||xpclib/Digital
  | Input/National
  | Instruments/PCI-MIO-16XE-10 ||__slNewName__||xpcnilib/Digital
  | Input/PCI-6030E ||__slOldName__||xpclib/Digital
  | Input/National
  | Instruments/PCI-6031E ||__slNewName__||xpcnilib/Digital
  | Input/PCI-6031E ||__slOldName__||xpclib/Digital
  | Input/National
  | Instruments/PXI-6527 ||__slNewName__||xpcnilib/Digital
  | Input/PXI-6527 ||__slOldName__||xpclib/Digital
  | Input/National
  | Instruments/PXI-6070E ||__slNewName__||xpcnilib/Digital
  | Input/PXI-6070E ||__slOldName__||xpclib/Digital
  | Input/National
  | Instruments/PXI-6040E ||__slNewName__||xpcnilib/Digital
  | Input/PXI-6040E ||__slOldName__||xpclib/Digital
  | Input/National
  | Instruments/PXI-6508 ||__slNewName__||xpcnilib/Digital
  | Input/PXI-6508 ||__slOldName__||xpclib/Digital
  | Input/National
  | Instruments/PXI-6071E ||__slNewName__||xpcnilib/Digital
  | Input/PXI-6071E ||__slOldName__||xpclib/Digital
  | Input/National
  | Instruments/PCI-6713 ||__slNewName__||xpcnilib/Digital
  | Input/PCI-6713 ||__slOldName__||xpclib/Digital
  | Input/National
  | Instruments/PXI-6713 ||__slNewName__||xpcnilib/Digital
  | Input/PXI-6713 ||__slOldName__||xpclib/Digital
  | Input/National
  | Instruments/PCI-6711 ||__slNewName__||xpcnilib/Digital
  | Input/PCI-6711 ||__slOldName__||xpclib/Digital
  | Input/Real Time
  | Devices/DM6420 ||__slNewName__||xpcrealtimedeviceslib/Digital
  | Input/DM6420 ||__slOldName__||xpclib/Digital
  | Input/Real Time
  | Devices/DM6430 ||__slNewName__||xpcrealtimedeviceslib/Digital
  | Input/DM6430 ||__slOldName__||xpclib/Digital
  | Input/Real Time
  | Devices/DM7420 ||__slNewName__||xpcrealtimedeviceslib/Digital
  | Input/DM7420 ||__slOldName__||xpclib/Digital
  | Input/Real Time
  | Devices/DM6604 ||__slNewName__||xpcrealtimedeviceslib/Digital
  | Input/DM6604 ||__slOldName__||xpclib/Digital
  | Input/Real Time
  | Devices/DM6804 ||__slNewName__||xpcrealtimedeviceslib/Digital
  | Input/DM6804 ||__slOldName__||xpclib/Digital
  | Input/Real Time
  | Devices/DM6814 ||__slNewName__||xpcrealtimedeviceslib/Digital
  | Input/DM6814 ||__slOldName__||xpclib/Digital
  | Input/SBS
  | Technologies/IP-Digital-24 ||__slNewName__||xpcsbstechnologieslib/Digital
  | Input/IP-Digital-24 ||__slOldName__||xpclib/Digital
  | Input/SBS
  | Technologies/IP-Unidig-E-48 ||__slNewName__||xpcsbstechnologieslib/Digital
  | Input/IP-Unidig-E-48 ||__slOldName__||xpclib/Digital
  | Input/UEI/PD2-MF 12bit series ||__slNewName__||xpcueilib/Digital
  | Input/PD2-MF 12bit series||__slOldName__||xpclib/Digital
  | Input/UEI/PD2-MFS 12bit series ||__slNewName__||xpcueilib/Digital
  | Input/PD2-MFS 12bit series||__slOldName__||xpclib/Digital
  | Input/UEI/PDXI-MF 12bit series ||__slNewName__||xpcueilib/Digital
  | Input/PDXI-MF 12bit series||__slOldName__||xpclib/Digital
  | Input/UEI/PDXI-MFS 12bit series ||__slNewName__||xpcueilib/Digital
  | Input/PDXI-MFS 12bit series||__slOldName__||xpclib/Digital
  | Input/UEI/PD2-MF 14bit series ||__slNewName__||xpcueilib/Digital
  | Input/PD2-MF 14bit series||__slOldName__||xpclib/Digital
  | Input/UEI/PD2-MFS 14bit series ||__slNewName__||xpcueilib/Digital
  | Input/PD2-MFS 14bit series||__slOldName__||xpclib/Digital
  | Input/UEI/PDXI-MF 14bit series ||__slNewName__||xpcueilib/Digital
  | Input/PDXI-MF 14bit series||__slOldName__||xpclib/Digital
  | Input/UEI/PDXI-MFS 14bit series ||__slNewName__||xpcueilib/Digital
  | Input/PDXI-MFS 14bit series||__slOldName__||xpclib/Digital
  | Input/UEI/PD2-MF 16bit series ||__slNewName__||xpcueilib/Digital
  | Input/PD2-MF 16bit series||__slOldName__||xpclib/Digital
  | Input/UEI/PD2-MFS 16bit series ||__slNewName__||xpcueilib/Digital
  | Input/PD2-MFS 16bit series||__slOldName__||xpclib/Digital
  | Input/UEI/PDXI-MF 16bit series ||__slNewName__||xpcueilib/Digital
  | Input/PDXI-MF 16bit series||__slOldName__||xpclib/Digital
  | Input/UEI/PDXI-MFS 16bit series ||__slNewName__||xpcueilib/Digital
  | Input/PDXI-MFS 16bit series||__slOldName__||xpclib/Digital
  | Input/UEI/PD2-AO series ||__slNewName__||xpcueilib/Digital
  | Input/PD2-AO series||__slOldName__||xpclib/Digital
  | Input/UEI/PDXI-AO series ||__slNewName__||xpcueilib/Digital
  | Input/PDXI-AO series||__slOldName__||xpclib/Digital
  | Input/Versalogic/VSBC-6 ||__slNewName__||xpcversalogiclib/Digital
  | Input/VSBC-6 ||__slOldName__||xpclib/Digital
  | Output/Advantech/PCL-711B||__slNewName__||xpcadvantechlib/Digital
  | Output/PCL-711B ||__slOldName__||xpclib/Digital
  | Output/Advantech/PCL-812||__slNewName__||xpcadvantechlib/Digital
  | Output/PCL-812 ||__slOldName__||xpclib/Digital
  | Output/Advantech/PCL-812PG||__slNewName__||xpcadvantechlib/Digital
  | Output/PCL-812PG ||__slOldName__||xpclib/Digital
  | Output/Advantech/PCL-818 ||__slNewName__||xpcadvantechlib/Digital
  | Output/PCL-818 ||__slOldName__||xpclib/Digital
  | Output/Advantech/PCL-818L ||__slNewName__||xpcadvantechlib/Digital
  | Output/PCL-818L ||__slOldName__||xpclib/Digital
  | Output/Advantech/PCL-818HG ||__slNewName__||xpcadvantechlib/Digital
  | Output/PCL-818HG ||__slOldName__||xpclib/Digital
  | Output/Advantech/PCL-818H ||__slNewName__||xpcadvantechlib/Digital
  | Output/PCL-818H ||__slOldName__||xpclib/Digital
  | Output/Advantech/PCL-818HD ||__slNewName__||xpcadvantechlib/Digital
  | Output/PCL-818HD ||__slOldName__||xpclib/Digital
  | Output/Advantech/PCL-1800 ||__slNewName__||xpcadvantechlib/Digital
  | Output/PCL-1800 ||__slOldName__||xpclib/Digital
  | Output/Advantech/PCL-726 ||__slNewName__||xpcadvantechlib/Digital
  | Output/PCL-726 ||__slOldName__||xpclib/Digital
  | Output/Advantech/PCL-727 ||__slNewName__||xpcadvantechlib/Digital
  | Output/PCL-727 ||__slOldName__||xpclib/Digital
  | Output/Analogic/AIM12 ||__slNewName__||xpcanalogiclib/Digital
  | Output/AIM12 ||__slOldName__||xpclib/Digital
  | Output/Analogic/AIM16 ||__slNewName__||xpcanalogiclib/Digital
  | Output/AIM16 ||__slOldName__||xpclib/Digital
  | Output/Burr-Brown/PCI-20041C ||__slNewName__||xpcobsoletelib/Burr-Brown/Digital
  | Output/PCI-20041C ||__slOldName__||xpclib/Digital
  | Output/Burr-Brown/PCI-20098C ||__slNewName__||xpcobsoletelib/Burr-Brown/Digital
  | Output/PCI-20098C ||__slOldName__||xpclib/Digital
  | Output/BVM/PMCDIO64 1||__slNewName__||xpcobsoletelib/BVM/Digital
  | Output/PMCDIO64 1 ||__slOldName__||xpclib/Digital
  | Output/Computer
  | Boards/CIO-DDA06 ||__slNewName__||xpcmeasurementcomputinglib/Digital
  | Output/CIO-DDA06 ||__slOldName__||xpclib/Digital
  | Output/Computer
  | Boards/CIO-DDA06//16 ||__slNewName__||xpcmeasurementcomputinglib/Digital
  | Output/CIO-DDA06//16 ||__slOldName__||xpclib/Digital
  | Output/Computer
  | Boards/CIO-DAS1601 12 ||__slNewName__||xpcmeasurementcomputinglib/Digital
  | Output/CIO-DAS1601 12 ||__slOldName__||xpclib/Digital
  | Output/Computer
  | Boards/CIO-DAS1602 12 ||__slNewName__||xpcmeasurementcomputinglib/Digital
  | Output/CIO-DAS1602 12 ||__slOldName__||xpclib/Digital
  | Output/Computer
  | Boards/CIO-DAS1602 16 ||__slNewName__||xpcmeasurementcomputinglib/Digital
  | Output/CIO-DAS1602 16 ||__slOldName__||xpclib/Digital
  | Output/Computer
  | Boards/CIO-DIO24 ||__slNewName__||xpcmeasurementcomputinglib/Digital
  | Output/CIO-DIO24 ||__slOldName__||xpclib/Digital
  | Output/Computer
  | Boards/CIO-DIO48 ||__slNewName__||xpcmeasurementcomputinglib/Digital
  | Output/CIO-DIO48 ||__slOldName__||xpclib/Digital
  | Output/Computer
  | Boards/CIO-DIO96 ||__slNewName__||xpcmeasurementcomputinglib/Digital
  | Output/CIO-DIO96 ||__slOldName__||xpclib/Digital
  | Output/Computer
  | Boards/CIO-DIO192 ||__slNewName__||xpcmeasurementcomputinglib/Digital
  | Output/CIO-DIO192 ||__slOldName__||xpclib/Digital
  | Output/Computer
  | Boards/CIO-DIO24H ||__slNewName__||xpcmeasurementcomputinglib/Digital
  | Output/CIO-DIO24H ||__slOldName__||xpclib/Digital
  | Output/Computer
  | Boards/CIO-DIO48H ||__slNewName__||xpcmeasurementcomputinglib/Digital
  | Output/CIO-DIO48H ||__slOldName__||xpclib/Digital
  | Output/Computer
  | Boards/CIO-PDISO16 ||__slNewName__||xpcmeasurementcomputinglib/Digital
  | Output/CIO-PDISO16 ||__slOldName__||xpclib/Digital
  | Output/Computer
  | Boards/CIO-DO24DD ||__slNewName__||xpcmeasurementcomputinglib/Digital
  | Output/CIO-DO24DD ||__slOldName__||xpclib/Digital
  | Output/Computer
  | Boards/PC104-DAS16JR 12 ||__slNewName__||xpcmeasurementcomputinglib/Digital
  | Output/PC104-DAS16JR 12 ||__slOldName__||xpclib/Digital
  | Output/Computer
  | Boards/PC104-DAS16JR 16 ||__slNewName__||xpcmeasurementcomputinglib/Digital
  | Output/PC104-DAS16JR 16 ||__slOldName__||xpclib/Digital
  | Output/Computer
  | Boards/PC104-DIO48 ||__slNewName__||xpcmeasurementcomputinglib/Digital
  | Output/PC104-DIO48 ||__slOldName__||xpclib/Digital
  | Output/Computer
  | Boards/PCI-DAS1200 ||__slNewName__||xpcmeasurementcomputinglib/Digital
  | Output/PCI-DAS1200 ||__slOldName__||xpclib/Digital
  | Output/Computer
  | Boards/PCI-DAS1200 JR ||__slNewName__||xpcmeasurementcomputinglib/Digital
  | Output/PCI-DAS1200 JR ||__slOldName__||xpclib/Digital
  | Output/Computer
  | Boards/PCI-DAS1602 12 ||__slNewName__||xpcmeasurementcomputinglib/Digital
  | Output/PCI-DAS1602 12 ||__slOldName__||xpclib/Digital
  | Output/Computer
  | Boards/PCI-DAS1602 16 ||__slNewName__||xpcmeasurementcomputinglib/Digital
  | Output/PCI-DAS1602 16 ||__slOldName__||xpclib/Digital
  | Output/Computer
  | Boards/PCIM-DAS1602 16 ||__slNewName__||xpcmeasurementcomputinglib/Digital
  | Output/PCIM-DAS1602 16 ||__slOldName__||xpclib/Digital
  | Output/Computer
  | Boards/PCI-DIO24 ||__slNewName__||xpcmeasurementcomputinglib/Digital
  | Output/PCI-DIO24 ||__slOldName__||xpclib/Digital
  | Output/Computer
  | Boards/PCI-DIO24H ||__slNewName__||xpcmeasurementcomputinglib/Digital
  | Output/PCI-DIO24H ||__slOldName__||xpclib/Digital
  | Output/Computer
  | Boards/PCI-DIO48H ||__slNewName__||xpcmeasurementcomputinglib/Digital
  | Output/PCI-DIO48H ||__slOldName__||xpclib/Digital
  | Output/Computer
  | Boards/PCI-DIO96 ||__slNewName__||xpcmeasurementcomputinglib/Digital
  | Output/PCI-DIO96 ||__slOldName__||xpclib/Digital
  | Output/Computer
  | Boards/PCI-DIO96H ||__slNewName__||xpcmeasurementcomputinglib/Digital
  | Output/PCI-DIO96H ||__slOldName__||xpclib/Digital
  | Output/Computer
  | Boards/PCI-DDA02 12 ||__slNewName__||xpcmeasurementcomputinglib/Digital
  | Output/PCI-DDA02 12 ||__slOldName__||xpclib/Digital
  | Output/Computer
  | Boards/PCI-DDA04 12 ||__slNewName__||xpcmeasurementcomputinglib/Digital
  | Output/PCI-DDA04 12 ||__slOldName__||xpclib/Digital
  | Output/Computer
  | Boards/PCI-DDA08 12 ||__slNewName__||xpcmeasurementcomputinglib/Digital
  | Output/PCI-DDA08 12 ||__slOldName__||xpclib/Digital
  | Output/Computer
  | Boards/PCI-PDISO8 ||__slNewName__||xpcmeasurementcomputinglib/Digital
  | Output/PCI-PDISO8 ||__slOldName__||xpclib/Digital
  | Output/Computer
  | Boards/PCI-PDISO16 ||__slNewName__||xpcmeasurementcomputinglib/Digital
  | Output/PCI-PDISO16 ||__slOldName__||xpclib/Digital
  | Output/Computer
  | Boards/PCI-DDA02 16 ||__slNewName__||xpcmeasurementcomputinglib/Digital
  | Output/PCI-DDA02 16 ||__slOldName__||xpclib/Digital
  | Output/Computer
  | Boards/PCI-DDA04 16 ||__slNewName__||xpcmeasurementcomputinglib/Digital
  | Output/PCI-DDA04 16 ||__slOldName__||xpclib/Digital
  | Output/Computer
  | Boards/PCI-DDA08 16 ||__slNewName__||xpcmeasurementcomputinglib/Digital
  | Output/PCI-DDA08 16 ||__slOldName__||xpclib/Digital
  | Output/Computer
  | Boards/PCIM-DDA06 16 ||__slNewName__||xpcmeasurementcomputinglib/Digital
  | Output/PCIM-DDA06 16 ||__slOldName__||xpclib/Digital
  | Output/Computer
  | Boards/PCI-DUAL-AC5 ||__slNewName__||xpcmeasurementcomputinglib/Digital
  | Output/PCI-DUAL-AC5 ||__slOldName__||xpclib/Digital
  | Output/Contec/PIO-3232T ||__slNewName__||xpcconteclib/Digital
  | Output/PIO-3232T ||__slOldName__||xpclib/Digital
  | Output/Contec/AD12-16  ||__slNewName__||xpcconteclib/Digital
  | Output/AD12-16 ||__slOldName__||xpclib/Digital
  | Output/Contec/AD12-64 ||__slNewName__||xpcconteclib/Digital
  | Output/AD12-64 ||__slOldName__||xpclib/Digital
  | Output/Data
  | Translation/DT2821 ||__slNewName__||xpcdatatranslationlib/Digital
  | Output/DT2821 ||__slOldName__||xpclib/Digital
  | Output/Data
  | Translation/DT2821-F-16SE ||__slNewName__||xpcdatatranslationlib/Digital
  | Output/DT2821-F-16SE ||__slOldName__||xpclib/Digital
  | Output/Data
  | Translation/DT2821-F-8DI ||__slNewName__||xpcdatatranslationlib/Digital
  | Output/DT2821-F-8DI ||__slOldName__||xpclib/Digital
  | Output/Data
  | Translation/DT2821-G-16SE ||__slNewName__||xpcdatatranslationlib/Digital
  | Output/DT2821-G-16SE ||__slOldName__||xpclib/Digital
  | Output/Data
  | Translation/DT2821-G-8DI ||__slNewName__||xpcdatatranslationlib/Digital
  | Output/DT2821-G-8DI ||__slOldName__||xpclib/Digital
  | Output/Data
  | Translation/DT2823 ||__slNewName__||xpcdatatranslationlib/Digital
  | Output/DT2823 ||__slOldName__||xpclib/Digital
  | Output/Data
  | Translation/DT2824-PGH ||__slNewName__||xpcdatatranslationlib/Digital
  | Output/DT2824-PGH ||__slOldName__||xpclib/Digital
  | Output/Data
  | Translation/DT2824-PGL ||__slNewName__||xpcdatatranslationlib/Digital
  | Output/DT2824-PGL ||__slOldName__||xpclib/Digital
  | Output/Data
  | Translation/DT2825 ||__slNewName__||xpcdatatranslationlib/Digital
  | Output/DT2825 ||__slOldName__||xpclib/Digital
  | Output/Data
  | Translation/DT2827 ||__slNewName__||xpcdatatranslationlib/Digital
  | Output/DT2827 ||__slOldName__||xpclib/Digital
  | Output/Data
  | Translation/DT2828 ||__slNewName__||xpcdatatranslationlib/Digital
  | Output/DT2828 ||__slOldName__||xpclib/Digital
  | Output/Diamond/Ruby-MM ||__slNewName__||xpcdiamondlib/Digital
  | Output/Ruby-MM ||__slOldName__||xpclib/Digital
  | Output/Diamond/Ruby-MM-416 ||__slNewName__||xpcdiamondlib/Digital
  | Output/Ruby-MM-416 ||__slOldName__||xpclib/Digital
  | Output/Diamond/Ruby-MM-1612 ||__slNewName__||xpcdiamondlib/Digital
  | Output/Ruby-MM-1612 ||__slOldName__||xpclib/Digital
  | Output/Diamond/QUARTZ-MM-5 ||__slNewName__||xpcdiamondlib/Digital
  | Output/QUARTZ-MM-5 ||__slOldName__||xpclib/Digital
  | Output/Diamond/QUARTZ-MM-10 ||__slNewName__||xpcdiamondlib/Digital
  | Output/QUARTZ-MM-10 ||__slOldName__||xpclib/Digital
  | Output/Diamond/Prometheus ||__slNewName__||xpcdiamondlib/Digital
  | Output/Prometheus||__slOldName__||xpclib/Digital
  | Output/Diamond/MM ||__slNewName__||xpcdiamondlib/Digital
  | Output/MM ||__slOldName__||xpclib/Digital
  | Output/Diamond/MM-32 ||__slNewName__||xpcdiamondlib/Digital
  | Output/MM-32 ||__slOldName__||xpclib/Digital
  | Output/Diamond/MM-16-AT ||__slNewName__||xpcdiamondlib/Digital
  | Output/MM-16-AT ||__slOldName__||xpclib/Digital
  | Output/Diamond/Onyx-MM ||__slNewName__||xpcdiamondlib/Digital
  | Output/Onyx-MM ||__slOldName__||xpclib/Digital
  | Output/Diamond/Onyx-MM-DIO ||__slNewName__||xpcdiamondlib/Digital
  | Output/Onyx-MM-DIO ||__slOldName__||xpclib/Digital
  | Output/Diamond/Garnet-MM ||__slNewName__||xpcdiamondlib/Digital
  | Output/Garnet-MM ||__slOldName__||xpclib/Digital
  | Output/General
  | Standards/ADADIO  ||__slNewName__||xpcgeneralstandardslib/Digital
  | Output/ADADIO ||__slOldName__||xpclib/Digital
  | Output/Gespac/GESPIA-2A ||__slNewName__||xpcobsoletelib/Gespac/Digital
  | Output/GESPIA-2A ||__slOldName__||xpclib/Digital
  | Output/Humusoft/AD 512 ||__slNewName__||xpchumusoftlib/Digital
  | Output/AD 512 ||__slOldName__||xpclib/Digital
  | Output/Keithley
  | Metrabyte/KPCI-1801HC ||__slNewName__||xpckeithleylib/Digital
  | Output/KPCI-1801HC ||__slOldName__||xpclib/Digital
  | Output/Keithley
  | Metrabyte/KPCI-1802HC  ||__slNewName__||xpckeithleylib/Digital
  | Output/KPCI-1802HC ||__slOldName__||xpclib/Digital
  | Output/Keithley
  | Metrabyte/DAS-1800HR ||__slNewName__||xpckeithleylib/Digital
  | Output/DAS-1800HR ||__slOldName__||xpclib/Digital
  | Output/National
  | Instruments/PC-DIO-24 ||__slNewName__||xpcnilib/Digital
  | Output/PC-DIO-24 ||__slOldName__||xpclib/Digital
  | Output/National
  | Instruments/PC-TIO-10 ||__slNewName__||xpcnilib/Digital
  | Output/PC-TIO-10 ||__slOldName__||xpclib/Digital
  | Output/National
  | Instruments/PCI-6503 ||__slNewName__||xpcnilib/Digital
  | Output/PCI-6503 ||__slOldName__||xpclib/Digital
  | Output/National
  | Instruments/PCI-DIO-96 ||__slNewName__||xpcnilib/Digital
  | Output/PCI-DIO-96 ||__slOldName__||xpclib/Digital
  | Output/National
  | Instruments/PCI-6023E ||__slNewName__||xpcnilib/Digital
  | Output/PCI-6023E ||__slOldName__||xpclib/Digital
  | Output/National
  | Instruments/PCI-6024E ||__slNewName__||xpcnilib/Digital
  | Output/PCI-6024E ||__slOldName__||xpclib/Digital
  | Output/National
  | Instruments/PCI-6025E ||__slNewName__||xpcnilib/Digital
  | Output/PCI-6025E ||__slOldName__||xpclib/Digital
  | Output/National
  | Instruments/PCI-6025E 8255 ||__slNewName__||xpcnilib/Digital
  | Output/PCI-6025E 8255 ||__slOldName__||xpclib/Digital
  | Output/National
  | Instruments/PCI-MIO-16E-1 ||__slNewName__||xpcnilib/Digital
  | Output/PCI-6070E ||__slOldName__||xpclib/Digital
  | Output/National
  | Instruments/PCI-MIO-16E-4 ||__slNewName__||xpcnilib/Digital
  | Output/PCI-6040E ||__slOldName__||xpclib/Digital
  | Output/National
  | Instruments/PCI-6071E ||__slNewName__||xpcnilib/Digital
  | Output/PCI-6071E ||__slOldName__||xpclib/Digital
  | Output/National
  | Instruments/PCI-6527 ||__slNewName__||xpcnilib/Digital
  | Output/PCI-6527 ||__slOldName__||xpclib/Digital
  | Output/National
  | Instruments/PCI-6052E ||__slNewName__||xpcnilib/Digital
  | Output/PCI-6052E ||__slOldName__||xpclib/Digital
  | Output/National
  | Instruments/PCI-MIO-16XE-10 ||__slNewName__||xpcnilib/Digital
  | Output/PCI-6030E ||__slOldName__||xpclib/Digital
  | Output/National
  | Instruments/PCI-6031E ||__slNewName__||xpcnilib/Digital
  | Output/PCI-6031E ||__slOldName__||xpclib/Digital
  | Output/National
  | Instruments/PXI-6527 ||__slNewName__||xpcnilib/Digital
  | Output/PXI-6527 ||__slOldName__||xpclib/Digital
  | Output/National
  | Instruments/PXI-6070E ||__slNewName__||xpcnilib/Digital
  | Output/PXI-6070E ||__slOldName__||xpclib/Digital
  | Output/National
  | Instruments/PXI-6040E ||__slNewName__||xpcnilib/Digital
  | Output/PXI-6040E ||__slOldName__||xpclib/Digital
  | Output/National
  | Instruments/PXI-6508 ||__slNewName__||xpcnilib/Digital
  | Output/PXI-6508 ||__slOldName__||xpclib/Digital
  | Output/National
  | Instruments/PXI-6071E ||__slNewName__||xpcnilib/Digital
  | Output/PXI-6071E ||__slOldName__||xpclib/Digital
  | Output/National
  | Instruments/PCI-6713 ||__slNewName__||xpcnilib/Digital
  | Output/PCI-6713 ||__slOldName__||xpclib/Digital
  | Output/National
  | Instruments/PXI-6713 ||__slNewName__||xpcnilib/Digital
  | Output/PXI-6713 ||__slOldName__||xpclib/Digital
  | Output/National
  | Instruments/PCI-6711 ||__slNewName__||xpcnilib/Digital
  | Output/PCI-6711 ||__slOldName__||xpclib/Digital
  | Output/Real Time
  | Devices/DM6420 ||__slNewName__||xpcrealtimedeviceslib/Digital
  | Output/DM6420 ||__slOldName__||xpclib/Digital
  | Output/Real Time
  | Devices/DM6430 ||__slNewName__||xpcrealtimedeviceslib/Digital
  | Output/DM6430 ||__slOldName__||xpclib/Digital
  | Output/Real Time
  | Devices/DM7420 ||__slNewName__||xpcrealtimedeviceslib/Digital
  | Output/DM7420 ||__slOldName__||xpclib/Digital
  | Output/Real Time
  | Devices/DM6604  ||__slNewName__||xpcrealtimedeviceslib/Digital
  | Output/DM6604 ||__slOldName__||xpclib/Digital
  | Output/Real Time
  | Devices/DM6804 ||__slNewName__||xpcrealtimedeviceslib/Digital
  | Output/DM6804 ||__slOldName__||xpclib/Digital
  | Output/Real Time
  | Devices/DM6814 ||__slNewName__||xpcrealtimedeviceslib/Digital
  | Output/DM6814 ||__slOldName__||xpclib/Digital
  | Output/SBS
  | Technologies
  | /IP-Digital-24||__slNewName__||xpcsbstechnologieslib/Digital
  | Output/IP-Digital-24 ||__slOldName__||xpclib/Digital
  | Output/SBS
  | Technologies
  | /IP-Unidig-E-48||__slNewName__||xpcsbstechnologieslib/Digital
  | Output/IP-Unidig-E-48 ||__slOldName__||xpclib/Digital
  | Output/UEI/PD2-MF 12bit series ||__slNewName__||xpcueilib/Digital
  | Output/PD2-MF 12bit series||__slOldName__||xpclib/Digital
  | Output/UEI/PD2-MFS 12bit series ||__slNewName__||xpcueilib/Digital
  | Output/PD2-MFS 12bit series||__slOldName__||xpclib/Digital
  | Output/UEI/PDXI-MF 12bit series ||__slNewName__||xpcueilib/Digital
  | Output/PDXI-MF 12bit series||__slOldName__||xpclib/Digital
  | Output/UEI/PDXI-MFS 12bit series ||__slNewName__||xpcueilib/Digital
  | Output/PDXI-MFS 12bit series||__slOldName__||xpclib/Digital
  | Output/UEI/PD2-MF 14bit series ||__slNewName__||xpcueilib/Digital
  | Output/PD2-MF 14bit series||__slOldName__||xpclib/Digital
  | Output/UEI/PD2-MFS 14bit series ||__slNewName__||xpcueilib/Digital
  | Output/PD2-MFS 14bit series||__slOldName__||xpclib/Digital
  | Output/UEI/PDXI-MF 14bit series ||__slNewName__||xpcueilib/Digital
  | Output/PDXI-MF 14bit series||__slOldName__||xpclib/Digital
  | Output/UEI/PDXI-MFS 14bit series ||__slNewName__||xpcueilib/Digital
  | Output/PDXI-MFS 14bit series||__slOldName__||xpclib/Digital
  | Output/UEI/PD2-MF 16bit series ||__slNewName__||xpcueilib/Digital
  | Output/PD2-MF 16bit series||__slOldName__||xpclib/Digital
  | Output/UEI/PD2-MFS 16bit series ||__slNewName__||xpcueilib/Digital
  | Output/PD2-MFS 16bit series||__slOldName__||xpclib/Digital
  | Output/UEI/PDXI-MF 16bit series ||__slNewName__||xpcueilib/Digital
  | Output/PDXI-MF 16bit series||__slOldName__||xpclib/Digital
  | Output/UEI/PDXI-MFS 16bit series ||__slNewName__||xpcueilib/Digital
  | Output/PDXI-MFS 16bit series||__slOldName__||xpclib/Digital
  | Output/UEI/PD2-AO series ||__slNewName__||xpcueilib/Digital
  | Output/PD2-AO series||__slOldName__||xpclib/Digital
  | Output/UEI/PDXI-AO series ||__slNewName__||xpcueilib/Digital
  | Output/PDXI-AO series||__slOldName__||xpclib/Digital
  | Output/Versalogic/VSBC-6 ||__slNewName__||xpcversalogiclib/Digital
  | Output/VSBC-6 ||__slOldName__||xpclib/Counter/Computer
  | Boards/CIO-CTRxx ||__slNewName__||xpcmeasurementcomputinglib/Counter/CIO-CTRxx ||__slOldName__||xpclib/Counter/Computer
  | Boards/CIO-CTR05 ||__slNewName__||xpcmeasurementcomputinglib/Counter/CIO-CTR05 ||__slOldName__||xpclib/Counter/Computer
  | Boards/CIO-CTR05 1||__slNewName__||xpcmeasurementcomputinglib/Counter/CIO-CTR05 1||__slOldName__||xpclib/Counter/Computer
  | Boards/CIO-CTR05 2||__slNewName__||xpcmeasurementcomputinglib/Counter/CIO-CTR05 2||__slOldName__||xpclib/Counter/Computer
  | Boards/CIO-CTR05 3||__slNewName__||xpcmeasurementcomputinglib/Counter/CIO-CTR05 3||__slOldName__||xpclib/Counter/Computer
  | Boards/CIO-CTR05 4||__slNewName__||xpcmeasurementcomputinglib/Counter/CIO-CTR05 4||__slOldName__||xpclib/Counter/Computer
  | Boards/CIO-CTR05 5||__slNewName__||xpcmeasurementcomputinglib/Counter/CIO-CTR05 5||__slOldName__||xpclib/Counter/Computer
  | Boards/CIO-CTR10 ||__slNewName__||xpcmeasurementcomputinglib/Counter/CIO-CTR10 ||__slOldName__||xpclib/Counter/Computer
  | Boards/CIO-CTR10 1||__slNewName__||xpcmeasurementcomputinglib/Counter/CIO-CTR10 1||__slOldName__||xpclib/Counter/Computer
  | Boards/CIO-CTR10 2||__slNewName__||xpcmeasurementcomputinglib/Counter/CIO-CTR10 2||__slOldName__||xpclib/Counter/Computer
  | Boards/CIO-CTR10 3||__slNewName__||xpcmeasurementcomputinglib/Counter/CIO-CTR10 3||__slOldName__||xpclib/Counter/Computer
  | Boards/CIO-CTR10 4||__slNewName__||xpcmeasurementcomputinglib/Counter/CIO-CTR10 4||__slOldName__||xpclib/Counter/Computer
  | Boards/CIO-CTR10 5||__slNewName__||xpcmeasurementcomputinglib/Counter/CIO-CTR10 5||__slOldName__||xpclib/Counter/Computer
  | Boards/PCI-CTR05  ||__slNewName__||xpcmeasurementcomputinglib/Counter/PCI-CTR05  ||__slOldName__||xpclib/Counter/Computer
  | Boards/PCI-CTR05 ||__slNewName__||xpcmeasurementcomputinglib/Counter/PCI-CTR05 ||__slOldName__||xpclib/Counter/Computer
  | Boards/PCI-CTR05 1||__slNewName__||xpcmeasurementcomputinglib/Counter/PCI-CTR05 1||__slOldName__||xpclib/Counter/Computer
  | Boards/PCI-CTR05 2||__slNewName__||xpcmeasurementcomputinglib/Counter/PCI-CTR05 2||__slOldName__||xpclib/Counter/Computer
  | Boards/PCI-CTR05 3||__slNewName__||xpcmeasurementcomputinglib/Counter/PCI-CTR05 3||__slOldName__||xpclib/Counter/Computer
  | Boards/PCI-CTR05 4||__slNewName__||xpcmeasurementcomputinglib/Counter/PCI-CTR05 4||__slOldName__||xpclib/Counter/Computer
  | Boards/PCI-CTR05 5||__slNewName__||xpcmeasurementcomputinglib/Counter/PCI-CTR05 5||__slOldName__||xpclib/Counter/Diamond/QUARTZ-MM ||__slNewName__||xpcdiamondlib/Counter/QUARTZ-MM ||__slOldName__||xpclib/Counter/Diamond/QUARTZ-MM-5 ||__slNewName__||xpcdiamondlib/Counter/QUARTZ-MM-5 ||__slOldName__||xpclib/Counter/Diamond/QUARTZ-MM-5 1||__slNewName__||xpcdiamondlib/Counter/QUARTZ-MM-5 1||__slOldName__||xpclib/Counter/Diamond/QUARTZ-MM-5 2||__slNewName__||xpcdiamondlib/Counter/QUARTZ-MM-5 2||__slOldName__||xpclib/Counter/Diamond/QUARTZ-MM-5 3||__slNewName__||xpcdiamondlib/Counter/QUARTZ-MM-5 3||__slOldName__||xpclib/Counter/Diamond/QUARTZ-MM-5 4||__slNewName__||xpcdiamondlib/Counter/QUARTZ-MM-5 4||__slOldName__||xpclib/Counter/Diamond/QUARTZ-MM-5 5||__slNewName__||xpcdiamondlib/Counter/QUARTZ-MM-5 5||__slOldName__||xpclib/Counter/Diamond/QUARTZ-MM-10 ||__slNewName__||xpcdiamondlib/Counter/QUARTZ-MM-10 ||__slOldName__||xpclib/Counter/Diamond/QUARTZ-MM-10 1||__slNewName__||xpcdiamondlib/Counter/QUARTZ-MM-10 1||__slOldName__||xpclib/Counter/Diamond/QUARTZ-MM-10 2||__slNewName__||xpcdiamondlib/Counter/QUARTZ-MM-10 2||__slOldName__||xpclib/Counter/Diamond/QUARTZ-MM-10 3||__slNewName__||xpcdiamondlib/Counter/QUARTZ-MM-10 3||__slOldName__||xpclib/Counter/Diamond/QUARTZ-MM-10 4||__slNewName__||xpcdiamondlib/Counter/QUARTZ-MM-10 4||__slOldName__||xpclib/Counter/Diamond/QUARTZ-MM-10 5||__slNewName__||xpcdiamondlib/Counter/QUARTZ-MM-10 5||__slOldName__||xpclib/Counter/National
  | Instruments/PC-TIO-xx ||__slNewName__||xpcnilib/Counter/PC-TIO-xx ||__slOldName__||xpclib/Counter/National
  | Instruments/PC-TIO-10 ||__slNewName__||xpcnilib/Counter/PC-TIO-10 ||__slOldName__||xpclib/Counter/National
  | Instruments/PC-TIO-10 1||__slNewName__||xpcnilib/Counter/PC-TIO-10 1||__slOldName__||xpclib/Counter/National
  | Instruments/PC-TIO-10 2||__slNewName__||xpcnilib/Counter/PC-TIO-10 2||__slOldName__||xpclib/Counter/National
  | Instruments/PC-TIO-10 3||__slNewName__||xpcnilib/Counter/PC-TIO-10 3||__slOldName__||xpclib/Counter/National
  | Instruments/PC-TIO-10 4||__slNewName__||xpcnilib/Counter/PC-TIO-10 4||__slOldName__||xpclib/Counter/National
  | Instruments/PC-TIO-10 5||__slNewName__||xpcnilib/Counter/PC-TIO-10 5||__slOldName__||xpclib/Counter/National
  | Instruments/PCI-6023E ||__slNewName__||xpcnilib/Counter/PCI-6023E ||__slOldName__||xpclib/Counter/National
  | Instruments/PCI-6024E ||__slNewName__||xpcnilib/Counter/PCI-6024E ||__slOldName__||xpclib/Counter/National
  | Instruments/PCI-6025E ||__slNewName__||xpcnilib/Counter/PCI-6025E ||__slOldName__||xpclib/Counter/National
  | Instruments/PCI-MIO-16E-1 ||__slNewName__||xpcnilib/Counter/PCI-6070E ||__slOldName__||xpclib/Counter/National
  | Instruments/PCI-MIO-16E-4 ||__slNewName__||xpcnilib/Counter/PCI-6040E ||__slOldName__||xpclib/Counter/National
  | Instruments/PXI-6070E ||__slNewName__||xpcnilib/Counter/PXI-6070E ||__slOldName__||xpclib/Counter/National
  | Instruments/PXI-6040E ||__slNewName__||xpcnilib/Counter/PXI-6040E ||__slOldName__||xpclib/Counter/National
  | Instruments/PCI-6071E ||__slNewName__||xpcnilib/Counter/PCI-6071E ||__slOldName__||xpclib/Counter/National
  | Instruments/PCI-6052E ||__slNewName__||xpcnilib/Counter/PCI-6052E ||__slOldName__||xpclib/Counter/National
  | Instruments/PCI-MIO-16XE-10 ||__slNewName__||xpcnilib/Counter/PCI-6030E ||__slOldName__||xpclib/Counter/National
  | Instruments/PCI-6031E ||__slNewName__||xpcnilib/Counter/PCI-6031E ||__slOldName__||xpclib/Counter/National
  | Instruments/PXI-6071E ||__slNewName__||xpcnilib/Counter/PXI-6071E ||__slOldName__||xpclib/Counter/National
  | Instruments/PCI-6023E 1||__slNewName__||xpcnilib/Counter/PCI-6023E 1||__slOldName__||xpclib/Counter/National
  | Instruments/PCI-6024E 1||__slNewName__||xpcnilib/Counter/PCI-6024E 1||__slOldName__||xpclib/Counter/National
  | Instruments/PCI-6025E 1||__slNewName__||xpcnilib/Counter/PCI-6025E 1||__slOldName__||xpclib/Counter/National
  | Instruments/PCI-MIO-16E-1 1||__slNewName__||xpcnilib/Counter/PCI-6070E 1||__slOldName__||xpclib/Counter/National
  | Instruments/PCI-MIO-16E-4 1||__slNewName__||xpcnilib/Counter/PCI-6040E 1||__slOldName__||xpclib/Counter/National
  | Instruments/PXI-6070E 1||__slNewName__||xpcnilib/Counter/PXI-6070E 1||__slOldName__||xpclib/Counter/National
  | Instruments/PXI-6040E 1||__slNewName__||xpcnilib/Counter/PXI-6040E 1||__slOldName__||xpclib/Counter/National
  | Instruments/PCI-6071E 1||__slNewName__||xpcnilib/Counter/PCI-6071E 1||__slOldName__||xpclib/Counter/National
  | Instruments/PCI-6052E 1||__slNewName__||xpcnilib/Counter/PCI-6052E 1||__slOldName__||xpclib/Counter/National
  | Instruments/PCI-MIO-16XE-10 1||__slNewName__||xpcnilib/Counter/PCI-6030E 1||__slOldName__||xpclib/Counter/National
  | Instruments/PCI-6031E 1||__slNewName__||xpcnilib/Counter/PCI-6031E 1||__slOldName__||xpclib/Counter/National
  | Instruments/PXI-6071E 1||__slNewName__||xpcnilib/Counter/PXI-6071E 1||__slOldName__||xpclib/Counter/Real Time
  | Devices/DM6804 ||__slNewName__||xpcrealtimedeviceslib/Counter/DM6804 ||__slOldName__||xpclib/Counter/Real Time
  | Devices/DM6804 1||__slNewName__||xpcrealtimedeviceslib/Counter/DM6804 1||__slOldName__||xpclib/Counter/Real Time
  | Devices/DM6804 2||__slNewName__||xpcrealtimedeviceslib/Counter/DM6804 2||__slOldName__||xpclib/Counter/Real Time
  | Devices/DM6804 3||__slNewName__||xpcrealtimedeviceslib/Counter/DM6804 3||__slOldName__||xpclib/Counter/Real Time
  | Devices/DM6804 4||__slNewName__||xpcrealtimedeviceslib/Counter/DM6804 4||__slOldName__||xpclib/Counter/Real Time
  | Devices/DM6804 5||__slNewName__||xpcrealtimedeviceslib/Counter/DM6804 5||__slOldName__||xpclib/Counter/Real Time
  | Devices/DM6804 6||__slNewName__||xpcrealtimedeviceslib/Counter/DM6804 6||__slOldName__||xpclib/Counter/Real Time
  | Devices/DM6816 ||__slNewName__||xpcrealtimedeviceslib/Counter/DM6816 ||__slOldName__||xpclib/Incremental
  | Encoder/ADDI-DATA/PA-1700 ||__slNewName__||xpcaddidatalib/Incremental
  | Encoder/PA-1700 ||__slOldName__||xpclib/Incremental
  | Encoder/ADDI-DATA/APCI-1710 enc ||__slNewName__||xpcaddidatalib/Incremental
  | Encoder/APCI-1710 enc ||__slOldName__||xpclib/Incremental
  | Encoder/Computer
  | Boards/PCI-QUAD04  ||__slNewName__||xpcmeasurementcomputinglib/Incremental
  | Encoder/PCI-QUAD04 ||__slOldName__||xpclib/Incremental
  | Encoder/Computer
  | Boards/CIO-QUAD02  ||__slNewName__||xpcmeasurementcomputinglib/Incremental
  | Encoder/CIO-QUAD02 ||__slOldName__||xpclib/Incremental
  | Encoder/Computer
  | Boards/CIO-QUAD04 ||__slNewName__||xpcmeasurementcomputinglib/Incremental
  | Encoder/CIO-QUAD04 ||__slOldName__||xpclib/Incremental
  | Encoder/Computer
  | Boards/Obsolete
  | Drivers/PCI-QUAD04 obs ||__slNewName__||xpcobsoletelib/Measurement
  | Computing/Incremental
  | Encoder/PCI-QUAD04 obs||__slOldName__||xpclib/Incremental
  | Encoder/Computer
  | Boards/Obsolete
  | Drivers/CIO-QUAD02 obs ||__slNewName__||xpcobsoletelib/Measurement
  | Computing/Incremental
  | Encoder/CIO-QUAD02 obs||__slOldName__||xpclib/Incremental
  | Encoder/Computer
  | Boards/Obsolete
  | Drivers/CIO-QUAD04 obs ||__slNewName__||xpcobsoletelib/Measurement
  | Computing/Incremental
  | Encoder/CIO-QUAD04 obs||__slOldName__||xpclib/Incremental
  | Encoder/Contec/CNT24-4D ||__slNewName__||xpcconteclib/Incremental
  | Encoder/CNT24-4D ||__slOldName__||xpclib/Incremental
  | Encoder/National
  | Instruments/PCI-6601 ||__slNewName__||xpcnilib/Incremental
  | Encoder/PCI-6601 ||__slOldName__||xpclib/Incremental
  | Encoder/Real Time
  | Devices/DM6814 ||__slNewName__||xpcrealtimedeviceslib/Incremental
  | Encoder/DM6814 ||__slOldName__||xpclib/LVDT/NAII/73LD3 ||__slNewName__||xpcnaiilib/LVDT/73LD3 ||__slOldName__||xpclib/LVDT/NAII/76CL1 ||__slNewName__||xpcnaiilib/LVDT/76CL1 ||__slOldName__||xpclib/LVDT/NAII/76LD1 ||__slNewName__||xpcnaiilib/LVDT/76LD1 ||__slOldName__||xpclib/LVDT/NAII/76CL1 1||__slNewName__||xpcnaiilib/LVDT/76CL1 1||__slOldName__||xpclib/Synchro
  | Resolver/NAII/PC-12SD ||__slNewName__||xpcnaiilib/Synchro
  | Resolver/PC-12SD ||__slOldName__||xpclib/Synchro
  | Resolver/NAII/76CS1 ||__slNewName__||xpcnaiilib/Synchro
  | Resolver/76CS1 ||__slOldName__||xpclib/Synchro
  | Resolver/NAII/73SD3 ||__slNewName__||xpcnaiilib/Synchro
  | Resolver/73SD3 ||__slOldName__||xpclib/Synchro
  | Resolver/NAII/76CS1 1||__slNewName__||xpcnaiilib/Synchro
  | Resolver/76CS1 1||__slOldName__||xpclib/Synchro
  | Resolver/SBS
  |  Technologies/IP-Synchro ||__slNewName__||xpcsbstechnologieslib/Synchro
  | Resolver/IP-Synchro ||__slOldName__||xpclib/GPIB/National
  | Instruments/GPIB-232CT-A ||__slNewName__||xpcnilib/GPIB/GPIB-232CT-A ||__slOldName__||xpclib/GPIB/National
  | Instruments/GPIB-232CT-A 1||__slNewName__||xpcnilib/GPIB/GPIB-232CT-A 1||__slOldName__||xpclib/Thermo
  | couple/Computer
  | Boards/PCI-DAS-TC ||__slNewName__||xpcmeasurementcomputinglib/Thermo
  | couple/PCI-DAS-TC ||__slOldName__||xpclib/IP Carrier/PCI-40A  ||__slNewName__||xpcsbstechnologieslib/IP Carrier/PCI-40A ||__slOldName__||xpclib/IP Carrier/Flex-104A ||__slNewName__||xpcsbstechnologieslib/IP Carrier/Flex-104A ||__slOldName__||xpclib/Watchdog/Versalogic/VSBC-6 ||__slNewName__||xpcversalogiclib/Watchdog/VSBC-6
settings DataIOCC: SignalLoggingName=logsOut
settings OptimizationCC: BooleanDataType=off
settings DebuggingCC: CheckExecutionContextPreStartOutputMsg=on  CheckExecutionContextRuntimeOutputMsg=on  SolverPrmCheckMsg=none
settings HardwareCC: ProdHWDeviceType=Specified  TargetUnknown=on
settings SFSimCC: SFSimApplyToAllLibs=on  SFSimBuildMode=Incremental

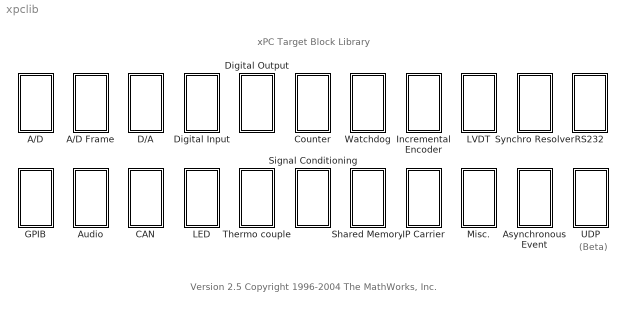
== system xpclib ==
  note: xPC Target Block Library
  note: Version 2.5
      | Copyright 1996-2004 The MathWorks, Inc.
  note: (Beta)
  A/D : Subsystem  PropExecContextAcrossSSBoundary=on
  A/D Frame : Subsystem  PropExecContextAcrossSSBoundary=on
  Asynchronous Event : Subsystem  PropExecContextAcrossSSBoundary=on
  Audio : Subsystem  PropExecContextAcrossSSBoundary=on
  CAN : Subsystem  PropExecContextAcrossSSBoundary=on
  Counter : Subsystem  PropExecContextAcrossSSBoundary=on
  D/A : Subsystem  PropExecContextAcrossSSBoundary=on
  Digital Input : Subsystem  PropExecContextAcrossSSBoundary=on
  Digital Output : Subsystem  PropExecContextAcrossSSBoundary=on
  GPIB : Subsystem  PropExecContextAcrossSSBoundary=on
  IP Carrier : Subsystem  InitFcn=mipcarrier  PropExecContextAcrossSSBoundary=on
  Incremental Encoder : Subsystem  PropExecContextAcrossSSBoundary=on
  LED : Subsystem  PropExecContextAcrossSSBoundary=on
  LVDT : Subsystem  PropExecContextAcrossSSBoundary=on
  Misc. : Subsystem  PropExecContextAcrossSSBoundary=on
  RS232 : Subsystem  PropExecContextAcrossSSBoundary=on
  Shared Memory : Subsystem  PropExecContextAcrossSSBoundary=on
  Signal Conditioning : Subsystem  PropExecContextAcrossSSBoundary=on
  Synchro Resolver : Subsystem  PropExecContextAcrossSSBoundary=on
  Thermo couple : Subsystem  PropExecContextAcrossSSBoundary=on
  UDP : Subsystem  PropExecContextAcrossSSBoundary=on
  Watchdog : Subsystem  InitFcn=mdacbpcidas(1);  PropExecContextAcrossSSBoundary=on
